simulink model "model"  (R2024b)
settings: Solver=ode4  StartTime=0.0  StopTime=1  FixedStep=0.0002  MaxStep=1e-4  RelTol=1e-3  EnableMultiTasking=on
values from neighbouring files (symbols this model uses):
  rr = 0.816    [lab2variables.m]
  rs = 0.435    [lab2variables.m]
  V_peak = (Vr_LL / sqrt(3)) * sqrt(2)    [lab2variables.m]
  w_b = 2 * pi * f_s    (= 376.991118431)    [lab2variables.m]
settings Model: PacingRate=0.200000  Creator=jw  LastModifiedBy=tnt4
settings SolverCC: AlgebraicLoopSolver=TrustRegion
settings DataIOCC: LimitDataPoints=on  SaveFormat=Array  SignalLoggingSaveFormat=ModelDataLogs  ReturnWorkspaceOutputs=off
settings OptimizationCC: InitFltsAndDblsToZero=on  LifeSpan=inf
settings DebuggingCC: SaveWithParameterizedLinksMsg=none  UnderspecifiedInitializationDetection=Classic  MergeDetectMultiDrivingBlocksExec=none  SignalResolutionControl=TryResolveAllWithWarning  SolverPrmCheckMsg=warning  MultiTaskDSMMsg=warning  MultiTaskCondExecSysMsg=none  FcnCallInpInsideContextMsg=warning  UnconnectedInputMsg=warning  UnconnectedOutputMsg=warning  UnconnectedLineMsg=warning  SFUnexpectedBacktrackingDiag=warning  SFNoUnconditionalDefaultTransitionDiag=warning  SFExecutionAtInitializationDiag=none  ArithmeticOperatorsInVariantConditions=warning
settings HardwareCC: ProdBitPerPointer=32  ProdBitPerSizeT=32  ProdBitPerPtrDiffT=32  ProdLargestAtomicFloat=None  ProdIntDivRoundTo=Undefined  ProdEndianess=Unspecified  ProdWordSize=32  ProdHWDeviceType=32-bit Generic
settings ModelReferenceCC: EnableRefExpFcnMdlSchedulingChecks=on  PropagateSignalLabelsOutOfModel=off
settings SFSimCC: SimUseLocalCustomCode=off  CustomCodeUndefinedFunction=UseInterfaceOnly
settings RTWCC: RTWUseLocalCustomCode=off  GPUComputeCapability=3.5
settings CodeAppCC: StateflowObjectComments=on
settings GRTTargetCC: TargetFcnLib=ansi_tfl_tmw.mat  TargetLangStandard=C89/C90 (ANSI)  CombineOutputUpdateFcns=off  GRTInterface=on
settings ConfigComp: CovMetricSettings=dw  CovSaveCumulativeToWorkspaceVar=on  CovSaveSingleToWorkspaceVar=on  CovExternalEMLEnable=off

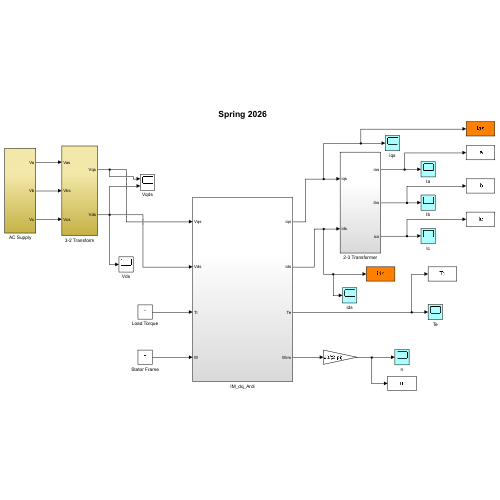
[thumbnail: Simulink's stored preview of the top-level diagram]
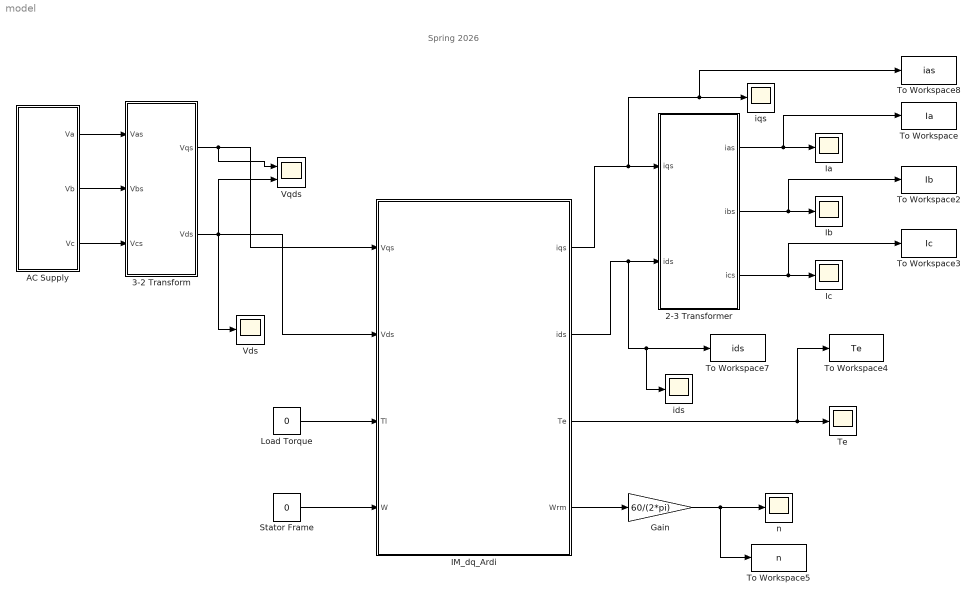
== system model ==
  note: Spring 2026
  2-3 Transformer : Subsystem
  3-2 Transform : Subsystem
  AC Supply : Subsystem  Description=g
  Gain : Gain  Gain=60/(2*pi)
  IM_dq_Ardi : Subsystem
  Ia : Scope
  Ib : Scope
  Ic : Scope
  Load Torque : Constant  Value=0
  Stator Frame : Constant  Value=0
  Te : Scope
  To Workspace : ToWorkspace  VariableName=Ia  SampleTime=-1
  To Workspace2 : ToWorkspace  VariableName=Ib  SampleTime=-1
  To Workspace3 : ToWorkspace  VariableName=Ic  SampleTime=-1
  To Workspace4 : ToWorkspace  VariableName=Te  SampleTime=-1
  To Workspace5 : ToWorkspace  VariableName=n  SampleTime=-1
  To Workspace7 : ToWorkspace  VariableName=ids  SampleTime=-1
  To Workspace8 : ToWorkspace  VariableName=ias  SampleTime=-1
  Vds : Scope
  Vqds : Scope  NumInputPorts=2
  ids : Scope
  iqs : Scope
  n : Scope
  wires:
  AC Supply/1(Va) -> 3-2 Transform/1(Vas)
  AC Supply/2(Vb) -> 3-2 Transform/2(Vbs)
  AC Supply/3(Vc) -> 3-2 Transform/3(Vcs)
  3-2 Transform/1(Vqs) -> Vqds/1, IM_dq_Ardi/1(Vqs)
  3-2 Transform/2(Vds) -> Vds/1, Vqds/2, IM_dq_Ardi/2(Vds)
  2-3 Transformer/1(ias) -> Ia/1, To Workspace/1
  2-3 Transformer/2(ibs) -> Ib/1, To Workspace2/1
  2-3 Transformer/3(ics) -> Ic/1, To Workspace3/1
  Load Torque/1 -> IM_dq_Ardi/3(Tl)
  Stator Frame/1 -> IM_dq_Ardi/4(W)
  IM_dq_Ardi/1(iqs) -> 2-3 Transformer/1(iqs), iqs/1, To Workspace8/1
  IM_dq_Ardi/2(ids) -> 2-3 Transformer/2(ids), ids/1, To Workspace7/1
  IM_dq_Ardi/4(Wrm) -> Gain/1
  Gain/1 -> n/1, To Workspace5/1
  IM_dq_Ardi/3(Te) -> Te/1, To Workspace4/1

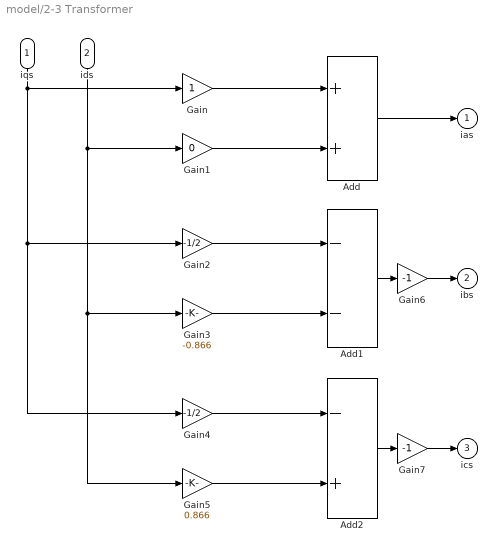
== system model/2-3 Transformer ==
  iqs : Inport
  ids : Inport  Port=2
  Add : Sum
  Add1 : Sum  Inputs=--
  Add2 : Sum  Inputs=-+
  Gain : Gain
  Gain1 : Gain  Gain=0
  Gain2 : Gain  Gain=-1/2
  Gain3 : Gain  Gain=-0.866
  Gain4 : Gain  Gain=-1/2
  Gain5 : Gain  Gain=0.866
  Gain6 : Gain  Gain=-1
  Gain7 : Gain  Gain=-1
  ias : Outport  InitialOutput=0  VectorParamsAs1DForOutWhenUnconnected=off
  ibs : Outport  Port=2  InitialOutput=0  VectorParamsAs1DForOutWhenUnconnected=off
  ics : Outport  Port=3  InitialOutput=0  VectorParamsAs1DForOutWhenUnconnected=off
  wires:
  Gain/1 -> Add/1
  Gain1/1 -> Add/2
  Gain2/1 -> Add1/1
  Gain3/1 -> Add1/2
  Gain4/1 -> Add2/1
  Gain5/1 -> Add2/2
  Add2/1 -> Gain7/1
  Add1/1 -> Gain6/1
  Add/1 -> ias/1
  iqs/1 -> Gain/1, Gain2/1, Gain4/1
  ids/1 -> Gain1/1, Gain3/1, Gain5/1
  Gain6/1 -> ibs/1
  Gain7/1 -> ics/1

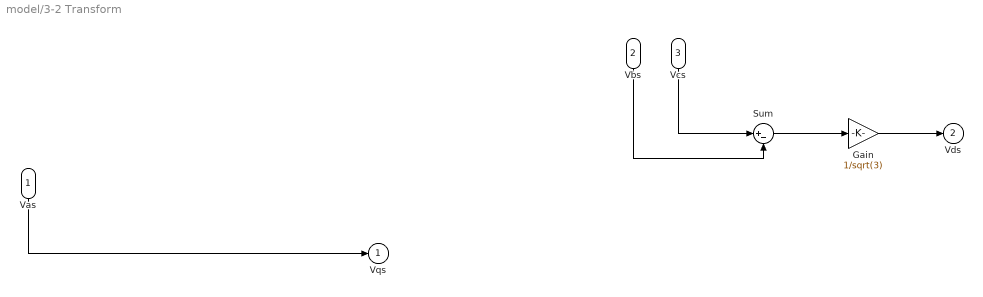
== system model/3-2 Transform ==
  Vas : Inport
  Vbs : Inport  Port=2
  Vcs : Inport  Port=3
  Gain : Gain  Gain=1/sqrt(3)
  Sum : Sum  Inputs=|+-
  Vqs : Outport  InitialOutput=0  VectorParamsAs1DForOutWhenUnconnected=off
  Vds : Outport  Port=2  InitialOutput=0  VectorParamsAs1DForOutWhenUnconnected=off
  wires:
  Vas/1 -> Vqs/1
  Vbs/1 -> Sum/2
  Vcs/1 -> Sum/1
  Sum/1 -> Gain/1
  Gain/1 -> Vds/1

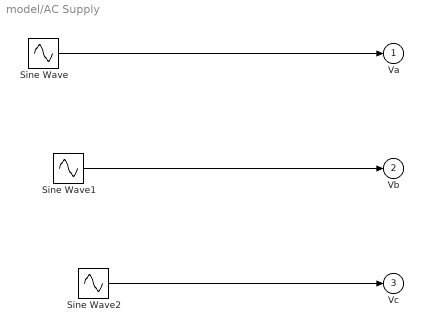
== system model/AC Supply ==
  Sine Wave : Sin  Amplitude=V_peak  Frequency=w_b  SampleTime=0
  Sine Wave1 : Sin  Amplitude=V_peak  Frequency=w_b  Phase=-2*pi/3  SampleTime=0
  Sine Wave2 : Sin  Amplitude=V_peak  Frequency=w_b  Phase=2*pi/3  SampleTime=0
  Va : Outport  InitialOutput=0  VectorParamsAs1DForOutWhenUnconnected=off
  Vb : Outport  Port=2  InitialOutput=0  VectorParamsAs1DForOutWhenUnconnected=off
  Vc : Outport  Port=3  InitialOutput=0  VectorParamsAs1DForOutWhenUnconnected=off
  wires:
  Sine Wave/1 -> Va/1
  Sine Wave1/1 -> Vb/1
  Sine Wave2/1 -> Vc/1

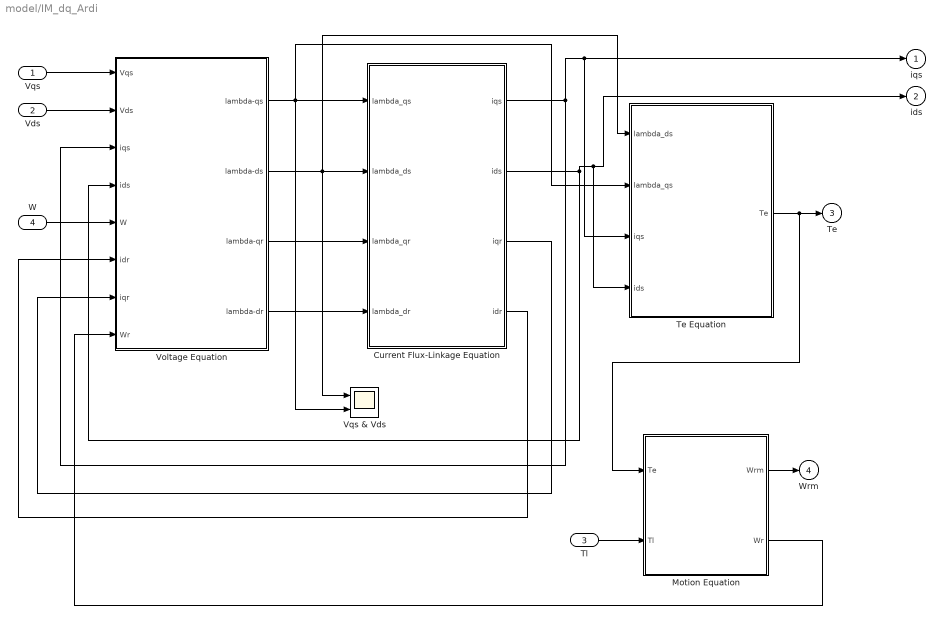
== system model/IM_dq_Ardi ==
  Vqs : Inport
  Vds : Inport  Port=2
  Tl : Inport  Port=3
  W : Inport  Port=4
  Current Flux-Linkage Equation : Subsystem
  Motion Equation : Subsystem
  Te Equation : Subsystem
  Voltage Equation : Subsystem
  Vqs & Vds : Scope  NumInputPorts=2
  iqs : Outport  InitialOutput=0  VectorParamsAs1DForOutWhenUnconnected=off
  ids : Outport  Port=2  InitialOutput=0  VectorParamsAs1DForOutWhenUnconnected=off
  Te : Outport  Port=3  InitialOutput=0  VectorParamsAs1DForOutWhenUnconnected=off
  Wrm : Outport  Port=4  InitialOutput=0  VectorParamsAs1DForOutWhenUnconnected=off
  wires:
  Vqs/1 -> Voltage Equation/1(Vqs)
  Vds/1 -> Voltage Equation/2(Vds)
  Tl/1 -> Motion Equation/2(Tl)
  W/1 -> Voltage Equation/5(W)
  Te Equation/1(Te) -> Te/1, Motion Equation/1(Te)
  Current Flux-Linkage Equation/1(iqs) -> Voltage Equation/3(iqs), iqs/1, Te Equation/3(iqs)
  Current Flux-Linkage Equation/2(ids) -> Voltage Equation/4(ids), ids/1, Te Equation/4(ids)
  Current Flux-Linkage Equation/3(iqr) -> Voltage Equation/7(iqr)
  Voltage Equation/1(lambda-qs) -> Vqs & Vds/2, Current Flux-Linkage Equation/1(lambda_qs), Te Equation/2(lambda_qs)
  Voltage Equation/2(lambda-ds) -> Te Equation/1(lambda_ds), Vqs & Vds/1, Current Flux-Linkage Equation/2(lambda_ds)
  Voltage Equation/3(lambda-qr) -> Current Flux-Linkage Equation/3(lambda_qr)
  Voltage Equation/4(lambda-dr) -> Current Flux-Linkage Equation/4(lambda_dr)
  Current Flux-Linkage Equation/4(idr) -> Voltage Equation/6(idr)
  Motion Equation/2(Wr) -> Voltage Equation/8(Wr)
  Motion Equation/1(Wrm) -> Wrm/1

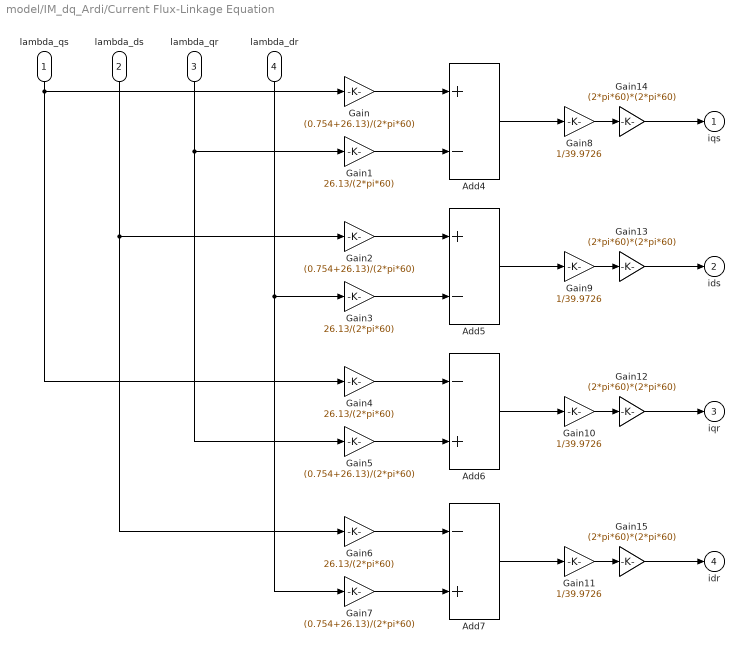
== system model/IM_dq_Ardi/Current Flux-Linkage Equation ==
  lambda_qs : Inport
  lambda_ds : Inport  Port=2
  lambda_qr : Inport  Port=3
  lambda_dr : Inport  Port=4
  Add4 : Sum  Inputs=+-
  Add5 : Sum  Inputs=+-
  Add6 : Sum  Inputs=-+
  Add7 : Sum  Inputs=-+
  Gain{,2,5,7} (4 alike) : Gain  Gain=(0.754+26.13)/(2*pi*60)
  Gain{1,3..4,6} (4 alike) : Gain  Gain=26.13/(2*pi*60)
  Gain{8..11} (4 alike) : Gain  Gain=1/39.9726
  Gain{12..15} (4 alike) : Gain  Gain=(2*pi*60)*(2*pi*60)
  iqs : Outport  InitialOutput=0  VectorParamsAs1DForOutWhenUnconnected=off
  ids : Outport  Port=2  InitialOutput=0  VectorParamsAs1DForOutWhenUnconnected=off
  iqr : Outport  Port=3  InitialOutput=0  VectorParamsAs1DForOutWhenUnconnected=off
  idr : Outport  Port=4  InitialOutput=0  VectorParamsAs1DForOutWhenUnconnected=off
  wires:
  Gain1/1 -> Add4/2
  Gain/1 -> Add4/1
  Gain2/1 -> Add5/1
  Gain3/1 -> Add5/2
  Gain4/1 -> Add6/1
  Gain5/1 -> Add6/2
  Gain6/1 -> Add7/1
  Gain7/1 -> Add7/2
  Add4/1 -> Gain8/1
  Add5/1 -> Gain9/1
  Add6/1 -> Gain10/1
  Add7/1 -> Gain11/1
  lambda_qs/1 -> Gain/1, Gain4/1
  lambda_qr/1 -> Gain1/1, Gain5/1
  Gain10/1 -> Gain12/1
  Gain9/1 -> Gain13/1
  Gain8/1 -> Gain14/1
  Gain11/1 -> Gain15/1
  lambda_ds/1 -> Gain2/1, Gain6/1
  lambda_dr/1 -> Gain3/1, Gain7/1
  Gain14/1 -> iqs/1
  Gain13/1 -> ids/1
  Gain12/1 -> iqr/1
  Gain15/1 -> idr/1

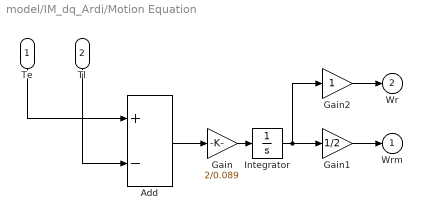
== system model/IM_dq_Ardi/Motion Equation ==
  Te : Inport
  Tl : Inport  Port=2
  Add : Sum  Inputs=+-
  Gain : Gain  Gain=2/0.089
  Gain1 : Gain  Gain=1/2
  Gain2 : Gain
  Integrator : Integrator
  Wrm : Outport  InitialOutput=0  VectorParamsAs1DForOutWhenUnconnected=off
  Wr : Outport  Port=2  InitialOutput=0  VectorParamsAs1DForOutWhenUnconnected=off
  wires:
  Te/1 -> Add/1
  Tl/1 -> Add/2
  Gain/1 -> Integrator/1
  Add/1 -> Gain/1
  Integrator/1 -> Gain2/1, Gain1/1
  Gain2/1 -> Wr/1
  Gain1/1 -> Wrm/1

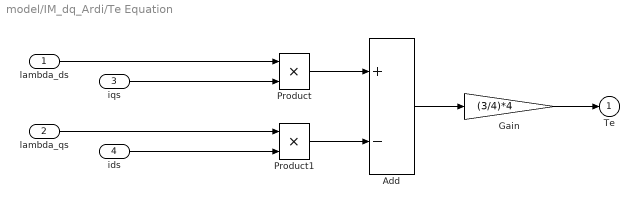
== system model/IM_dq_Ardi/Te Equation ==
  lambda_ds : Inport
  lambda_qs : Inport  Port=2
  iqs : Inport  Port=3
  ids : Inport  Port=4
  Add : Sum  Inputs=+-
  Gain : Gain  Gain=(3/4)*4
  Product : Product  RndMeth=Zero
  Product1 : Product  RndMeth=Zero
  Te : Outport  InitialOutput=0  VectorParamsAs1DForOutWhenUnconnected=off
  wires:
  Gain/1 -> Te/1
  Add/1 -> Gain/1
  lambda_ds/1 -> Product/1
  iqs/1 -> Product/2
  lambda_qs/1 -> Product1/1
  ids/1 -> Product1/2
  Product/1 -> Add/1
  Product1/1 -> Add/2

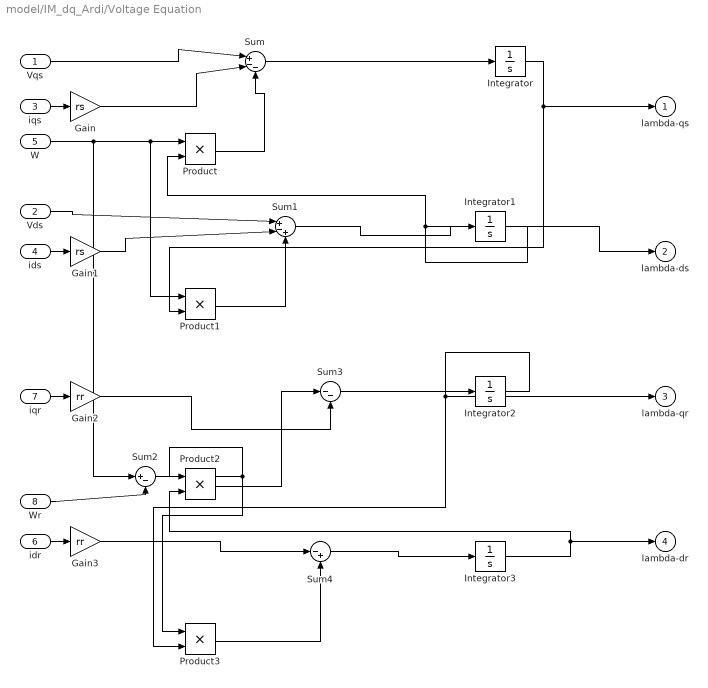
== system model/IM_dq_Ardi/Voltage Equation ==
  Vqs : Inport
  Vds : Inport  Port=2
  iqs : Inport  Port=3
  ids : Inport  Port=4
  W : Inport  Port=5
  idr : Inport  Port=6
  iqr : Inport  Port=7
  Wr : Inport  Port=8
  Gain : Gain  Gain=rs
  Gain1 : Gain  Gain=rs
  Gain2 : Gain  Gain=rr
  Gain3 : Gain  Gain=rr
  Integrator{,1..3} (4 alike) : Integrator
  Product{,1..3} (4 alike) : Product
  Sum : Sum  Inputs=|+--
  Sum1 : Sum  Inputs=|+-+
  Sum2 : Sum  Inputs=|+-
  Sum3 : Sum  Inputs=|--
  Sum4 : Sum  Inputs=|-+
  lambda-qs : Outport  InitialOutput=0  VectorParamsAs1DForOutWhenUnconnected=off
  lambda-ds : Outport  Port=2  InitialOutput=0  VectorParamsAs1DForOutWhenUnconnected=off
  lambda-qr : Outport  Port=3  InitialOutput=0  VectorParamsAs1DForOutWhenUnconnected=off
  lambda-dr : Outport  Port=4  InitialOutput=0  VectorParamsAs1DForOutWhenUnconnected=off
  wires:
  iqs/1 -> Gain/1
  Vqs/1 -> Sum/1
  Gain/1 -> Sum/2
  W/1 -> Sum2/1, Product1/1, Product/1
  Product/1 -> Sum/3
  Sum/1 -> Integrator/1
  Integrator/1 -> Product1/2, lambda-qs/1
  Vds/1 -> Sum1/1
  ids/1 -> Gain1/1
  Gain1/1 -> Sum1/2
  Product1/1 -> Sum1/3
  Sum1/1 -> Integrator1/1
  Integrator1/1 -> Product/2, lambda-ds/1
  Wr/1 -> Sum2/2
  iqr/1 -> Gain2/1
  Gain2/1 -> Sum3/2
  Sum2/1 -> Product3/1, Product2/1
  Product2/1 -> Sum3/1
  Sum3/1 -> Integrator2/1
  Integrator2/1 -> Product3/2, lambda-qr/1
  idr/1 -> Gain3/1
  Gain3/1 -> Sum4/1
  Product3/1 -> Sum4/2
  Integrator3/1 -> Product2/2, lambda-dr/1
  Sum4/1 -> Integrator3/1
